simulink model "control_system"  (R2021b)
settings: Solver=VariableStepAuto  StartTime=0.0  StopTime=10.0  RelTol=1e-3
undefined symbols (not defined in the file): k
settings Model: Creator=Richi  LastModifiedBy=Richi

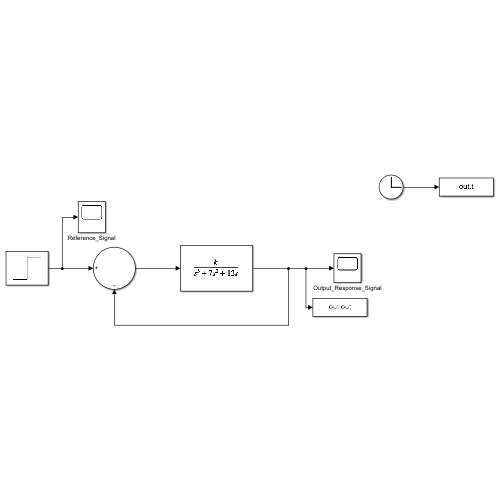
[thumbnail: Simulink's stored preview of the top-level diagram]
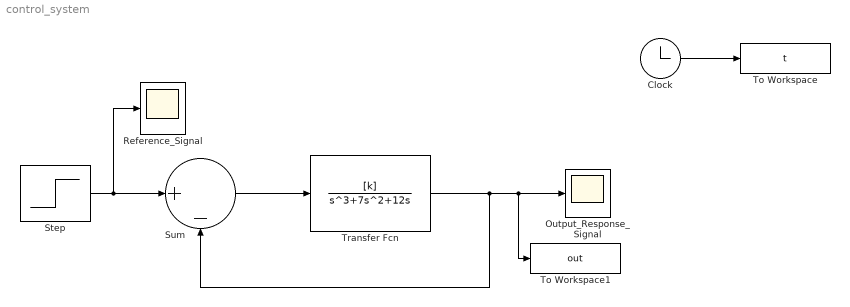
== system control_system ==
  Clock : Clock
  Output_Response_Signal : Scope
  Reference_Signal : Scope
  Step : Step  SampleTime=0
  Sum : Sum  Inputs=|+-
  To Workspace : ToWorkspace  VariableName=t  SaveFormat=Timeseries  SampleTime=-1
  To Workspace1 : ToWorkspace  VariableName=out  SaveFormat=Timeseries  SampleTime=-1
  Transfer Fcn : TransferFcn  Numerator=[k]  Denominator=[1 7 12 0]
  wires:
  Step/1 -> Reference_Signal/1, Sum/1
  Sum/1 -> Transfer Fcn/1
  Transfer Fcn/1 -> Sum/2, To Workspace1/1, Output_Response_Signal/1
  Clock/1 -> To Workspace/1
